simulink model "Ball_Bean_2016b"  (R2016b)
settings: Solver=ode4  StartTime=0.0  StopTime=200  FixedStep=0.05  RelTol=1e-3
model workspace (MAT data in the model file):
  k0 = Simulink.Parameter
  k0.DataType = 'auto'
  k0.Dimensions = [0 0]
undefined symbols (not defined in the file or in its folder): sigbuilder_block
libraries: fuzblock x1
settings Model: Creator=ASUS  LastModifiedBy=ASUS
settings DataIOCC: ReturnWorkspaceOutputs=on
settings SFSimCC: SimUseLocalCustomCode=on
settings RTWCC: RTWUseLocalCustomCode=on

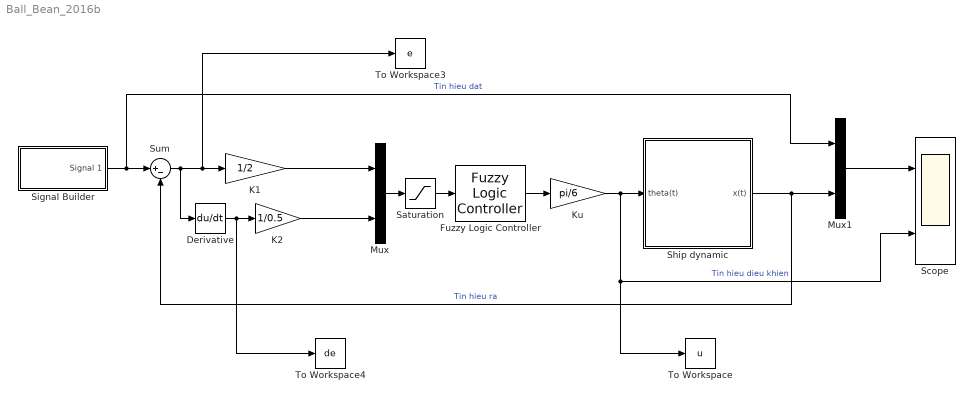
== system Ball_Bean_2016b ==
  Derivative : Derivative
  Fuzzy Logic Controller : fuzblock/Fuzzy Logic  Controller  FIS='bt3.fis'
  K1 : Gain  Gain=1/2
  K2 : Gain  Gain=1/0.5
  Ku : Gain  Gain=pi/6
  Mux : Mux  Inputs=2
  Mux1 : Mux  Inputs=2
  Saturation : Saturate  UpperLimit=1  LowerLimit=-1
  Scope : Scope  NumInputPorts=2
  Ship dynamic : Subsystem  mask{m=0.1, J=0.00005, R=0.02, g=9.81}
  Signal Builder : Subsystem  Tag=STV Subsys  LoadFcn=sigbuilder_block('load');  StartFcn=sigbuilder_block('start');  StopFcn=sigbuilder_block('stop');  ClipboardFcn=sigbuilder_block('clipboard');  mask(Sigbuilder block){tuvar=[0:10]}
      mask help: Simulink:masks:SigbuilderBlock_MD
      mask init:
      | if ~strcmp(get_param(bdroot(gcbh),'SimulationStatus'),'stopped') tuvar = sigbuilder_block('maskInit'); end
      settings: CopyFcn=sigbuilder_block('copy');  DeleteFcn=sigbuilder_block('delete');  ModelCloseFcn=sigbuilder_block('modelClose');  PreSaveFcn=sigbuilder_block('preSave');  PauseFcn=sigbuilder_block('pause');  ContinueFcn=sigbuilder_block('continue');  NameChangeFcn=sigbuilder_block('namechange');  OpenFcn=sigbuilder_block('open',[316.2 97.8 550.8 400.2 ]);  CloseFcn=sigbuilder_block('close');
      mask Display: plot(0, 0, 100, 100,[2, 2, 32, 32, 2], [68, 8, 8, 68, 68],[32, 2], [38, 38], [32, 19, 2],[53, 60, 44], [32, 17, 17, 2],[16, 16, 31, 31]);txt = getActiveGroup(gcbh);text(2, 100, txt,'verticalAlignment', 'top');
  Sum : Sum  Inputs=|+-
  To Workspace : ToWorkspace  VariableName=u  SampleTime=-1
  To Workspace3 : ToWorkspace  VariableName=e  SampleTime=-1
  To Workspace4 : ToWorkspace  VariableName=de  SampleTime=-1
  wires:
  Ku/1 -> To Workspace/1, Scope/2, Ship dynamic/1(theta(t))  "Tin hieu dieu khien"
  Fuzzy Logic Controller/1 -> Ku/1
  Saturation/1 -> Fuzzy Logic Controller/1
  Mux/1 -> Saturation/1
  Derivative/1 -> To Workspace4/1, K2/1
  K1/1 -> Mux/1
  K2/1 -> Mux/2
  Signal Builder/1(Signal 1) -> Mux1/1, Sum/1  "Tin hieu dat"
  Ship dynamic/1(x(t)) -> Sum/2, Mux1/2  "Tin hieu ra"
  Mux1/1 -> Scope/1
  Sum/1 -> To Workspace3/1, K1/1, Derivative/1

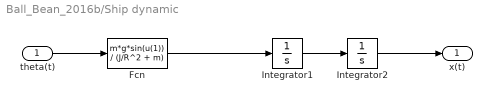
== system Ball_Bean_2016b/Ship dynamic ==
  theta(t) : Inport
  Fcn : Fcn  Expr=m*g*sin(u(1)) / (J/R^2 + m)
  Integrator1 : Integrator
  Integrator2 : Integrator
  x(t) : Outport
  wires:
  Integrator1/1 -> Integrator2/1
  Integrator2/1 -> x(t)/1
  Fcn/1 -> Integrator1/1
  theta(t)/1 -> Fcn/1

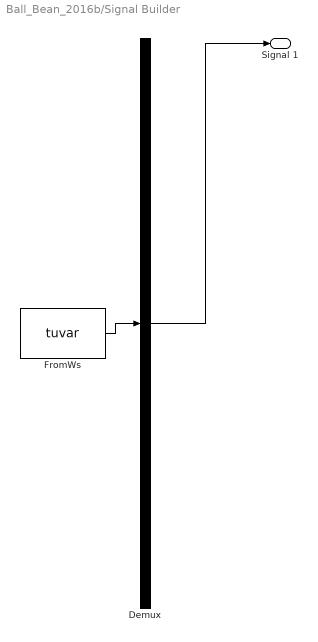
== system Ball_Bean_2016b/Signal Builder ==
  Demux : Demux  Tag=STV Demux  Outputs=1
  FromWs : FromWorkspace  Tag=STV FromWs  VariableName=tuvar  SampleTime=0
      SigBuilderData=|
      | common.afterFinalStr = 'Extrapolate'
      | common.sampleTime = 0
      | dataSet.timeRange = [0 200]
      | dataSet.name = 'Group 1'
      | sbobj.Groups.Name = 'Group 1'
      | sbobj.Groups.Signals.Name = 'Signal 1'
      | sbobj.Groups.Signals.XData = [0 11.5 11.5 26.5 26.5 42 42 62.5 62.5 87 87 108.5 108.5 137.5 137.5 165 165 187.5 187.5 200]
      | sbobj.Groups.Signals.YData = [-0.15 -0.15 0.915 0.915 -0.88 -0.88 0.915 0.915 -0.62 -0.62 -0.09 -0.09 0.32 0.32 0.915 0.915 0.12 0.12 -0.4 -0.4]
      | sbobj.Groups.TimeRange = [0 200]
  Signal 1 : Outport  Tag=STV Outport
  wires:
  Demux/1 -> Signal 1/1
  FromWs/1 -> Demux/1
